simulink model "main"  (R2019a)
settings: Solver=VariableStepAuto  StartTime=0.0  StopTime=1.5  RelTol=1e-3
model workspace: external: MATLAB File D:\Vs\New\iiwa_DataFile.m (data not in the file)
undefined symbols (not defined in the file or in its folder): smiData, X, Y, Z
libraries: sm_lib x49, nesl_utility x19, simulink x7, sharedtransform x1
(part 2 of 2)

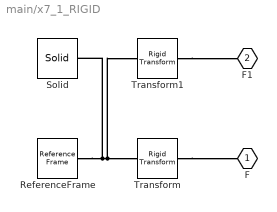
== system main/x7_1_RIGID ==
  ReferenceFrame : sm_lib/Frames and Transforms/Reference Frame
  Solid : sm_lib/Body Elements/Solid  InertiaType=Custom  Mass=2  MassUnits=kg  CenterOfMass=smiData.Solid(3).CoM  CenterOfMassUnits=mm  MomentsOfInertia=smiData.Solid(3).MoI  MomentsOfInertiaUnits=kg*mm^2  ProductsOfInertia=smiData.Solid(3).PoI  ProductsOfInertiaUnits=kg*mm^2  BasedOnType=Density  Density=1000  DensityUnits=kg/m^3  DoExposeReferenceFrame=on  SerializedFrames=<Frames/>  GraphicType=FromGeometry  MarkerShape=Sphere  MarkerSize=10  GraphicVisPropType=SimpleVisualProperties  GraphicDiffuseColor=smiData.Solid(3).color  GraphicSpecularColor=[0.5 0.5 0.5 1.0]  GraphicAmbientColor=[0.15 0.15 0.15 1.0]  GraphicEmissiveColor=[0.0 0.0 0.0 1.0]  GraphicShininess=75  GraphicOpacity=smiData.Solid(3).opacity  GeometryShape=FromFile  RectangleSize=[1 1]  RectangleSizeUnits=m  BrickDimensions=[1 1 1]  BrickDimensionUnits=m  CylinderRadius=1  CylinderRadiusUnits=m  CylinderLength=1  CylinderLengthUnits=m  SphereRadius=1  SphereRadiusUnits=m  EllipsoidRadii=[1 1 1]  EllipsoidRadiiUnits=m  ExtrusionCrossSection=[1 1; -1 1; -1 -1; 1 -1]  ExtrusionCrossSectionUnits=m  ExtrusionLength=1  ExtrusionLengthUnits=m  PolygonNumSides=3  PolygonOuterRadius=1  PolygonOuterRadiusUnits=m  ExtGeomFileType=STEP  ExtGeomFileName=7_Default_sldprt.STEP  ExtGeomFileUnits=m  RevolutionCrossSection=[1 1; 1 -1; 2 -1; 2 1]  RevolutionCrossSectionUnits=m  RevolutionExtent=Full  RevolutionAngle=180  RevolutionAngleUnits=deg
  Transform : sm_lib/Frames and Transforms/Rigid Transform  TranslationMethod=Cartesian  TranslationStandardOffset=0  TranslationLengthUnit=mm  TranslationStandardAxis=+Z  TranslationCartesianOffset=smiData.RigidTransform(12).translation  TranslationROffset=0  TranslationROffsetUnits=m  TranslationZOffset=0  TranslationZOffsetUnits=m  TranslationThetaOffset=0  TranslationThetaOffsetUnits=deg  RotationMethod=ArbitraryAxis  RotationAngleUnits=rad  RotationStandardAxis=+Z  RotationAngle=smiData.RigidTransform(12).angle  RotationArbitraryAxis=smiData.RigidTransform(12).axis  FollAlignAxisA=+X  BaseAlignAxisA=+Y  FollAlignAxisB=+Y  BaseAlignAxisB=+Z  RotationSequenceAxes=FollowerAxes  RotationSequence=XYX  RotationSequenceAngles=[0 0 0]  RotationSequenceAnglesUnits=deg  RotationMatrix=[1 0 0; 0 1 0; 0 0 1]
  Transform1 : sm_lib/Frames and Transforms/Rigid Transform  TranslationMethod=Cartesian  TranslationStandardOffset=0  TranslationLengthUnit=mm  TranslationStandardAxis=+Z  TranslationCartesianOffset=smiData.RigidTransform(13).translation  TranslationROffset=0  TranslationROffsetUnits=m  TranslationZOffset=0  TranslationZOffsetUnits=m  TranslationThetaOffset=0  TranslationThetaOffsetUnits=deg  RotationMethod=ArbitraryAxis  RotationAngleUnits=rad  RotationStandardAxis=+Z  RotationAngle=smiData.RigidTransform(13).angle  RotationArbitraryAxis=smiData.RigidTransform(13).axis  FollAlignAxisA=+X  BaseAlignAxisA=+Y  FollAlignAxisB=+Y  BaseAlignAxisB=+Z  RotationSequenceAxes=FollowerAxes  RotationSequence=XYX  RotationSequenceAngles=[0 0 0]  RotationSequenceAnglesUnits=deg  RotationMatrix=[1 0 0; 0 1 0; 0 0 1]
  F : PMIOPort  Side=Left
  F1 : PMIOPort  Port=2  Side=Right
  connections:
  Solid/RConn1 -- ReferenceFrame/RConn1 -- Transform/LConn1 -- Transform1/LConn1
  Transform/RConn1 -- F/RConn1
  Transform1/RConn1 -- F1/RConn1

== matlab function main/MATLAB Function1 ==
  data: q1 input; eef_transform output; J output; x output; y output; z output; q2 input; q3 input; q4 input; q5 input; q6 input; q7 input; rot output
function [eef_transform,J,x,y,z,rot]=directKinematics(q1,q2,q3,q4,q5,q6,q7)

% DH PARAMETERS FOR THE ROBOT
alfa={0,-pi/2,pi/2,pi/2,-pi/2,-pi/2,pi/2};

q=[q1,q2,q3,q4,q5,q6,q7];
% following are "d" parameters for iiwa 14 R 820 
%d={0.0,0.0,0.42,0.0,0.4,0.0,0.0};
d={0.36,0.0,0.42,0.0,0.4,0.0,0.126};

% The following is for accounting for the length of the flange "Medien-Flansch Touch pneumatisch".
d{7}=0.020+0.051; % if you have another type of flange, please refer to reference [1] above.
a={0,0,0,0,0,0,0};

%% Calculating the direct Kinematics
T=zeros(4,4,7);
i=1;
T(:,:,i)=getDHMatrix(alfa{i},q(i),d{i},a{i});
    for i=2:7
        T(:,:,i)=T(:,:,i-1)*getDHMatrix(alfa{i},q(i),d{i},a{i});
        T(:,:,i)=normalizeColumns(T(:,:,i));
    end
        T(:,:,7)=T(:,:,7);
        T(:,:,7)=normalizeColumns(T(:,:,7));
        
    pef=T(1:3,4,7);
    J=zeros(6,7);
    for i=1:7
        k=T(1:3,3,i);
        pij=pef-T(1:3,4,i);
        J(1:3,i)=cross(k,pij);
        J(4:6,i)=k;
    end
%% End effector transform
eef_transform=T(:,:,7);
x=T(1,4,7);
y=T(2,4,7);
z=T(3,4,7);
rot=T(1:3,1:3,7);
end

function T=getDHMatrix(alfa,theta,d,a)
T=zeros(4,4);
calpha=cos(alfa);
sinalpha=sin(alfa);
coshteta=cos(theta);
sintheta=sin(theta);

T(1,1)=coshteta;
T(2,1)=sintheta*calpha;
T(3,1)=sintheta*sinalpha;				

T(1,2)=-sintheta;
T(2,2)=coshteta*calpha;
T(3,2)=coshteta*sinalpha;

T(2,3)=-sinalpha;
T(3,3)=calpha;

T(1,4)=a;
T(2,4)=-sinalpha*d;
T(3,4)=calpha*d;
T(4,4)=1;

end

function normalizedT=normalizeColumns(T)
%% This function is used to normalize the columns of a rotation matrix with 
% some numerical errors resulting from matrix multiplication problems
r=zeros(4,3); % corrected rotatio matrix, with zero badding row at the end
for j=1:3
    r(1:3,j)=T(1:3,j)/norm(T(1:3,j));
end
normalizedT=[r,T(:,4)];
end

== matlab function main/MATLAB Function2 ==
  data: Pos input; q output; J input
function  q=directKinematics(Pos, J)

q=pinv(J)*Pos;

end

== matlab function main/MATLAB Function3 ==
function VisualServo()

    global A3D B3D C3D D3D A B C D Ad Bd Cd Dd

    %coordinates of the 4 points wrt camera frame
    A3D = [-0.2633;0.27547;0.8956];
    B3D = [0.2863;-0.2749;0.8937];
    C3D = [-0.2637;-0.2746;0.8977];
    D3D = [0.2866;0.2751;0.8916];

    %initial projections (computed here only to show their relation with the desired ones) 
    A=A3D(1:2)/A3D(3);
    B=B3D(1:2)/B3D(3);
    C=C3D(1:2)/C3D(3);
    D=D3D(1:2)/D3D(3);

    %initial camera position and orientation
    %orientation is expressed in Euler angles (X-Y-Z around the inertial frame
    %of reference)
    cam=[0;0;0;0;0;0];

    %desired projections
    Ad=A+[0.1;0];
    Bd=B;
    Cd=C+[0.1;0];
    Dd=D;

    t0 = 0;
    tf = 50;

    s0 = cam;

    %time step
    dt=0.01;
    t = euler_ode(t0, tf, dt, s0);

end


function ts = euler_ode(t0,tf,dt,s0)

    global A3D B3D C3D D3D Ad Bd Cd Dd 

    s = s0;
    ts=[];
    for t=t0:dt:tf
        ts(end+1)=t;
        cam = s;

        % rotation matrix R_WCS_CCS
        R = calc_Rotation_matrix(cam(4),cam(5),cam(6));
        r = cam(1:3);

        % 3D coordinates of the 4 points wrt the NEW camera frame
        A3D_cam = R'*(A3D-r);
        B3D_cam = R'*(B3D-r);
        C3D_cam = R'*(C3D-r);
        D3D_cam = R'*(D3D-r);

        % NEW projections
        A=A3D_cam(1:2)/A3D_cam(3);
        B=B3D_cam(1:2)/B3D_cam(3);
        C=C3D_cam(1:2)/C3D_cam(3);
        D=D3D_cam(1:2)/D3D_cam(3);


        % computing the L matrices
        L1 = L_matrix(A(1),A(2),A3D_cam(3));
        L2 = L_matrix(B(1),B(2),B3D_cam(3));
        L3 = L_matrix(C(1),C(2),C3D_cam(3));
        L4 = L_matrix(D(1),D(2),D3D_cam(3));
        L = [L1;L2;L3;L4];


        %updating the projection errors
        e = [A-Ad;B-Bd;C-Cd;D-Dd];

        %compute camera velocity
        vc = -0.5*pinv(L)*e;

        %change of the camera position and orientation
        ds = vc;

        %update camera position and orientation
        s = s + ds*dt;
    %cam = cam*expm(vc*dt)

    end  
    ts(end+1)=tf+dt;
end

function R = calc_Rotation_matrix(theta_x, theta_y, theta_z)

    Rx = [1 0 0; 0 cos(theta_x) -sin(theta_x); 0 sin(theta_x) cos(theta_x)];
    Ry = [cos(theta_y) 0 sin(theta_y); 0 1 0; -sin(theta_y) 0 cos(theta_y)];
    Rz = [cos(theta_z) -sin(theta_z) 0; sin(theta_z) cos(theta_z) 0; 0 0 1];

    R = Rx*Ry*Rz;

end

function L = L_matrix(x,y,z)

    L = [-1/z,0,x/z,x*y,-(1+x^2),y;
       0,-1/z,y/z,1+y^2,-x*y,-x];
end

== matlab function main/MATLAB Function4 ==
  data: R input; res output
function res=rot2eulZYX(R)
    [res]=eulerAngles(R) ;
end

function y=closeEnough(a,b)
    epsilon=0.000001;
    if (epsilon>abs(a-b))
        y=1;
    else
        y=0;
    end
end

function [res]=eulerAngles(R) 
    %% check for gimbal lock
    R=R';
    if (closeEnough(R(1,3), -1.0)) 
        b = 0; %% gimbal lock, value of x doesn't matter
        c = pi / 2;
        a = b + atan2(R(2,1), R(3,1));
    elseif (closeEnough(R(1,3), 1.0)) 
        b = 0;
        c = -pi / 2;
        a = -b + atan2(-R(2,1), -R(3,1));
    else  %% two solutions exist
        b1 = -asin(R(1,3));
        b2 = pi - b1;

        c1 = atan2(R(2,3) / cos(b1), R(3,3) / cos(b1));
        c2 = atan2(R(2,3) / cos(b2), R(3,3) / cos(b2));

        a1 = atan2(R(1,2) / cos(b1), R(1,1)/ cos(b1));
        a2 = atan2(R(1,2) / cos(b2), R(1,1) / cos(b2));

        %% choose one solution to return
        %% for example the "shortest" rotation
        condition=((abs(b1) + abs(c1) + abs(a1)) <= (abs(b2) + abs(c2) + abs(a2)));
        if condition 
            a=a1;
            b=b1;
            c=c1;   
        else 
            a=a2;
            b=b2;
            c=c2;   
        end
    end
    res=[a,b,c];
end
